simulink subsystem "Fault_Tolerant_Controller"  (R2022b)
settings: Solver=VariableStepAuto  StartTime=0.0  StopTime=10.0  RelTol=1e-3
libraries: matrix_library x2
settings Model: Creator=hunter  LastModifiedBy=hunter

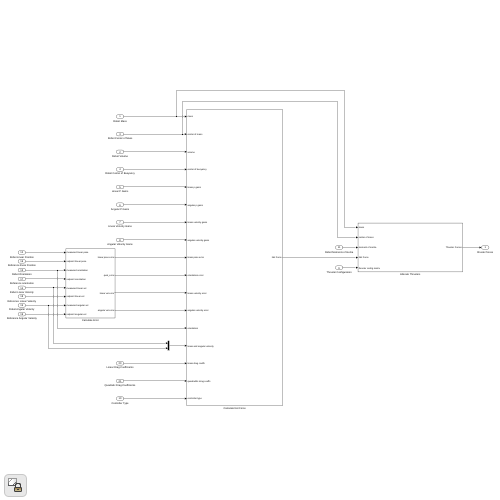
[thumbnail: Simulink's stored preview of the top-level diagram]
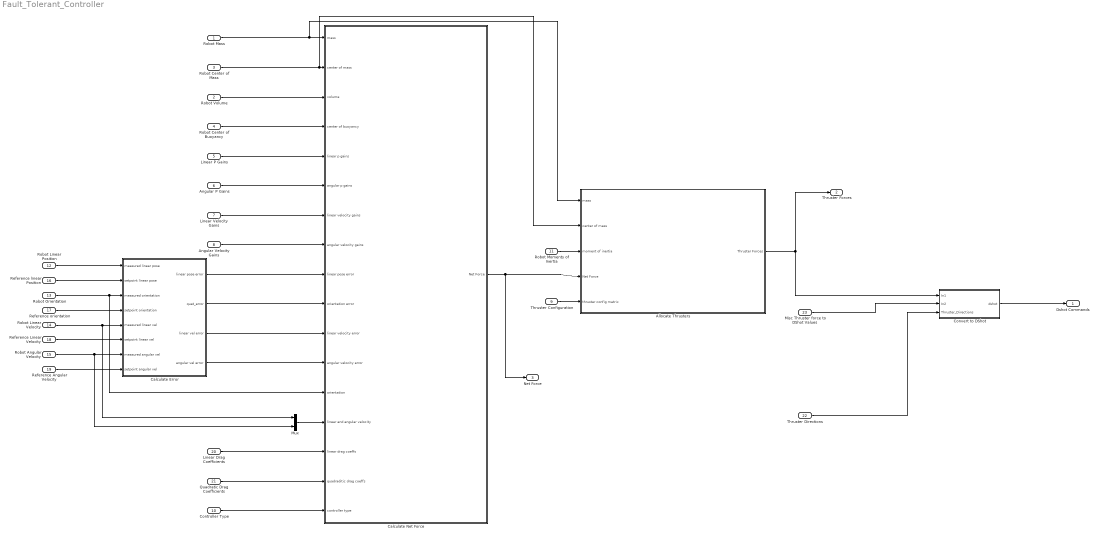
== system Fault_Tolerant_Controller ==
  Robot Mass : Inport  Unit=kg
  Robot Volume : Inport  Port=2  OutDataTypeStr=double
  Robot Center of Mass : Inport  Port=3  OutDataTypeStr=double  PortDimensions=[3 1]
  Robot Center of Buoyancy : Inport  Port=4  OutDataTypeStr=double  PortDimensions=[3 1]
  Linear P Gains : Inport  Port=5  OutDataTypeStr=double  PortDimensions=[3 3]
  Angular P Gains : Inport  Port=6  OutDataTypeStr=double  PortDimensions=[3 3]
  Linear Velocity Gains : Inport  Port=7  OutDataTypeStr=double  PortDimensions=[3 3]
  Angular Velocity Gains : Inport  Port=8  OutDataTypeStr=double  PortDimensions=[3 3]
  Thruster Configuration : Inport  Port=9  OutDataTypeStr=double  PortDimensions=[6 8]
  Controller Type : Inport  Port=10  OutDataTypeStr=boolean  PortDimensions=1
  Robot Moments of Inertia : Inport  Port=11  OutDataTypeStr=double  Unit=kg*m^2  PortDimensions=[3 1]
  Robot Linear Position : Inport  Port=12  OutDataTypeStr=double  PortDimensions=[3 1]
  Robot Orientation : Inport  Port=13  OutDataTypeStr=double  PortDimensions=[4 1]
  Robot Linear Velocity : Inport  Port=14  OutDataTypeStr=double  PortDimensions=[3 1]
  Robot Angular Velocity : Inport  Port=15  OutDataTypeStr=double  PortDimensions=[3 1]
  Reference linear Position : Inport  Port=16  OutDataTypeStr=double  PortDimensions=[3 1]
  Reference orientation : Inport  Port=17
  Reference Linear Velocity : Inport  Port=18
  Reference Angular Velocity : Inport  Port=19
  Linear Drag Coefficients : Inport  Port=20  OutDataTypeStr=double  PortDimensions=[6 1]
  Quadratic Drag Coefficients : Inport  Port=21  OutDataTypeStr=double  PortDimensions=[6 1]
  Thruster Directions : Inport  Port=22
  Misc Thruster force to DShot Values : Inport  Description=|  Port=23  OutDataTypeStr=double  PortDimensions=[11 1]
      | The rows of this column vector are defined as the following
      | Row 1 (C-style index 0): Max force for an individual thruster (max_force)
      | Row 2 (C-style index 1): Min force for and individual thruster (MIN_THRUST)
      | Row 3 (C-style index 2): Startup thrust force (STARTUP_THRUST)
      | 
      | Row 4 (C-style index 3): Positive slope for startup thrust (SU_THRUST.POS_SLOPE)
      | Row 5 (C-style index 4): Positive y-intercept for startup thrust (SU_THRUST.POS_YINT)
      | Row 6 (C-style index 5): Negative slope for startup thrust (SU_THRUST.NEG_SLOPE)
      | Row 7 (C-style index 6): Negative y-intercept for startup thrust (SU_THRUST.NEG_YINT)
      | 
      | Row 8 (C-style index 7): Positive slope for regular thrust (THRUST.POS_SLOPE)
      | Row 9 (C-style index 8): Positive y-intercept for regular thrust (THRUST.POS_YINT)
      | Row 10 (C-style index 9): Negative slope for regular thrust (THRUST.NEG_SLOPE)
      | Row 11 (C-style index 10): Negative y-intercept for regular thrust (THRUST.NEG_YINT)
      settings: AttributesFormatString=%<Description>
  Allocate Thrusters : Subsystem
  Calculate Error : Subsystem
  Calculate Net Force : Subsystem
  Convert to DShot : Subsystem
  Mux : Mux  Inputs=2
  Dshot Commands : Outport  OutDataTypeStr=int16  PortDimensions=[8 1]
  Thruster Forces : Outport  Port=2
  Net Force : Outport  Port=3
  wires:
  Robot Mass/1 -> Calculate Net Force/1(mass), Allocate Thrusters/1(mass)
  Robot Volume/1 -> Calculate Net Force/3(volume)
  Robot Center of Mass/1 -> Allocate Thrusters/2(center of mass), Calculate Net Force/2(center of mass)
  Robot Center of Buoyancy/1 -> Calculate Net Force/4(center of buoyancy)
  Linear P Gains/1 -> Calculate Net Force/5(linear p gains)
  Angular P Gains/1 -> Calculate Net Force/6(angular p gains)
  Linear Velocity Gains/1 -> Calculate Net Force/7(linear velocity gains)
  Angular Velocity Gains/1 -> Calculate Net Force/8(angular velocity gains)
  Controller Type/1 -> Calculate Net Force/17(controller type)
  Calculate Net Force/1(Net Force) -> Allocate Thrusters/4(Net Force), Net Force/1
  Thruster Configuration/1 -> Allocate Thrusters/5(thruster config matrix)
  Robot Moments of Inertia/1 -> Allocate Thrusters/3(moment of inertia)
  Robot Linear Position/1 -> Calculate Error/1(measured linear pose)
  Reference linear Position/1 -> Calculate Error/2(setpoint linear pose)
  Robot Orientation/1 -> Calculate Error/3(measured orientation), Calculate Net Force/13(orientation)
  Reference orientation/1 -> Calculate Error/4(setpoint orientation)
  Robot Linear Velocity/1 -> Calculate Error/5(measured linear vel), Mux/1
  Reference Linear Velocity/1 -> Calculate Error/6(setpoint linear vel)
  Robot Angular Velocity/1 -> Calculate Error/7(measured angular vel), Mux/2
  Reference Angular Velocity/1 -> Calculate Error/8(setpoint angular vel)
  Calculate Error/1(linear pose error) -> Calculate Net Force/9(linear pose error)
  Calculate Error/2(quat_error) -> Calculate Net Force/10(orientation error)
  Calculate Error/3(linear vel error) -> Calculate Net Force/11(linear velocity error)
  Calculate Error/4(angular vel error) -> Calculate Net Force/12(angular velocity error)
  Mux/1 -> Calculate Net Force/14(linear and angular velocity)
  Linear Drag Coefficients/1 -> Calculate Net Force/15(linear drag coeffs)
  Quadratic Drag Coefficients/1 -> Calculate Net Force/16(quadraditic drag coeffs)
  Allocate Thrusters/1(Thruster Forces) -> Convert to DShot/1(In1), Thruster Forces/1
  Misc Thruster force to DShot Values/1 -> Convert to DShot/2(In2)
  Thruster Directions/1 -> Convert to DShot/3(Thruster_Directions)
  Convert to DShot/1(dshot) -> Dshot Commands/1

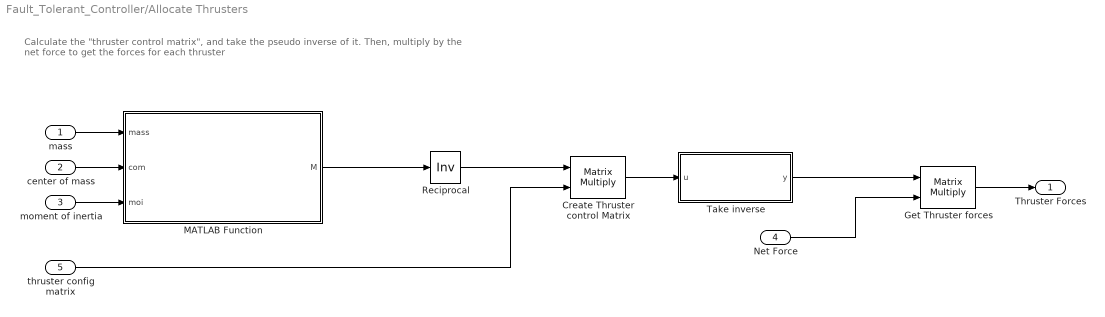
== system Fault_Tolerant_Controller/Allocate Thrusters ==
  note: Calculate the "thruster control matrix", and take the pseudo inverse of it.
      | Then, multiply by the net force to get the forces for each thruster
  mass : Inport
  center of mass : Inport  Port=2
  moment of inertia : Inport  Port=3
  Net Force : Inport  Port=4
  thruster config matrix : Inport  Port=5
  Create Thruster control Matrix : Product  Multiplication=Matrix(*)
  Get Thruster forces : Product  Multiplication=Matrix(*)
  MATLAB Function : MATLAB Function  TreatAsAtomicUnit=on
  Reciprocal : Product  Inputs=/  Multiplication=Matrix(*)
  Take inverse : MATLAB Function  TreatAsAtomicUnit=on
  Thruster Forces : Outport  OutDataTypeStr=double  PortDimensions=[8 1]
  wires:
  Get Thruster forces/1 -> Thruster Forces/1
  thruster config matrix/1 -> Create Thruster control Matrix/2
  Reciprocal/1 -> Create Thruster control Matrix/1
  Net Force/1 -> Get Thruster forces/2
  Take inverse/1(y) -> Get Thruster forces/1
  MATLAB Function/1(M) -> Reciprocal/1
  Create Thruster control Matrix/1 -> Take inverse/1(u)
  center of mass/1 -> MATLAB Function/2(com)
  moment of inertia/1 -> MATLAB Function/3(moi)
  mass/1 -> MATLAB Function/1(mass)

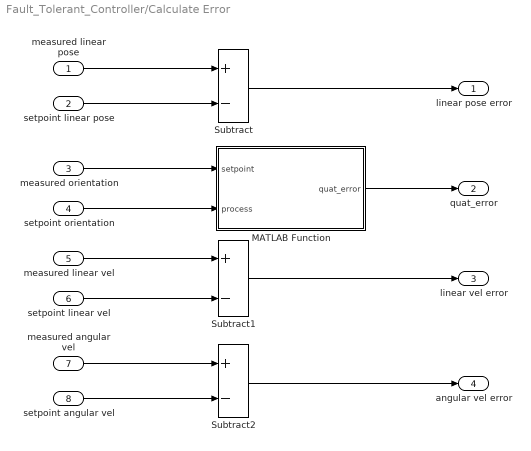
== system Fault_Tolerant_Controller/Calculate Error ==
  measured linear pose : Inport
  setpoint linear pose : Inport  Port=2
  measured orientation : Inport  Port=3
  setpoint orientation : Inport  Port=4  OutDataTypeStr=double  PortDimensions=[4 1]
  measured linear vel : Inport  Port=5
  setpoint linear vel : Inport  Port=6
  measured angular vel : Inport  Port=7
  setpoint angular vel : Inport  Port=8
  MATLAB Function : MATLAB Function  TreatAsAtomicUnit=on
  Subtract : Sum  Inputs=+-
  Subtract1 : Sum  Inputs=+-
  Subtract2 : Sum  Inputs=+-
  linear pose error : Outport
  quat_error : Outport  Port=2
  linear vel error : Outport  Port=3
  angular vel error : Outport  Port=4
  wires:
  setpoint angular vel/1 -> Subtract2/2
  measured angular vel/1 -> Subtract2/1
  measured linear vel/1 -> Subtract1/1
  setpoint linear vel/1 -> Subtract1/2
  setpoint linear pose/1 -> Subtract/2
  measured linear pose/1 -> Subtract/1
  Subtract/1 -> linear pose error/1
  Subtract1/1 -> linear vel error/1
  MATLAB Function/1(quat_error) -> quat_error/1
  Subtract2/1 -> angular vel error/1
  setpoint orientation/1 -> MATLAB Function/2(process)
  measured orientation/1 -> MATLAB Function/1(setpoint)

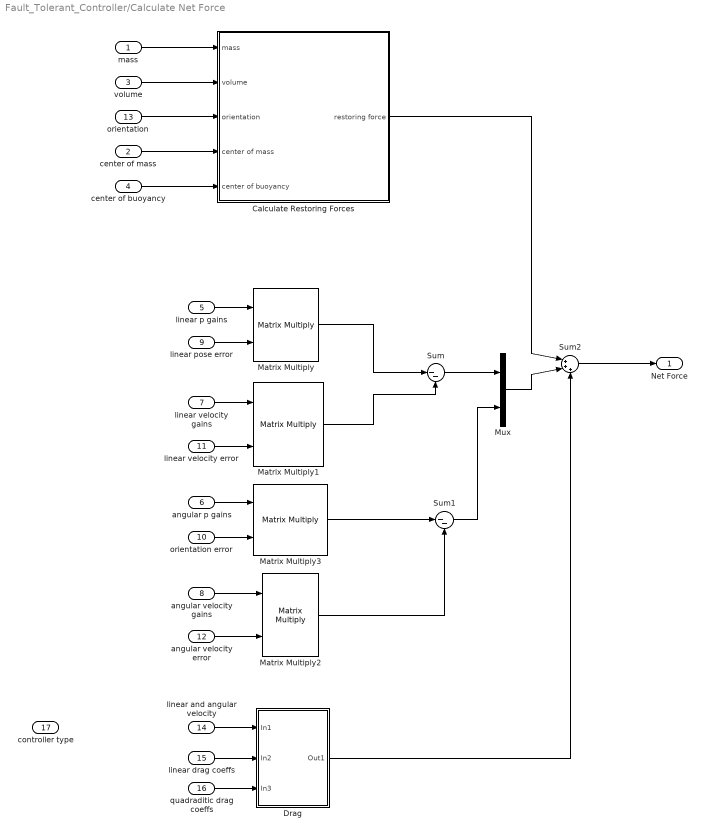
== system Fault_Tolerant_Controller/Calculate Net Force ==
  mass : Inport
  center of mass : Inport  Port=2
  volume : Inport  Port=3
  center of buoyancy : Inport  Port=4
  linear p gains : Inport  Port=5
  angular p gains : Inport  Port=6
  linear velocity gains : Inport  Port=7
  angular velocity gains : Inport  Port=8
  linear pose error : Inport  Port=9
  orientation error : Inport  Port=10
  linear velocity error : Inport  Port=11
  angular velocity error : Inport  Port=12
  orientation : Inport  Port=13
  linear and angular velocity : Inport  Port=14
  linear drag coeffs : Inport  Port=15
  quadraditic drag coeffs : Inport  Port=16
  controller type : Inport  Port=17
  Calculate Restoring Forces : Subsystem
  Drag : Subsystem
  Matrix Multiply{,1..3} (4 alike) : Product  Multiplication=Matrix(*)
  Mux : Mux  Inputs=2
  Sum : Sum  Inputs=|--
  Sum1 : Sum  Inputs=|--
  Sum2 : Sum  Inputs=|+++
  Net Force : Outport  OutDataTypeStr=double  Unit=N  PortDimensions=[6 1]
  wires:
  angular velocity gains/1 -> Matrix Multiply2/1
  angular velocity error/1 -> Matrix Multiply2/2
  angular p gains/1 -> Matrix Multiply3/1
  orientation error/1 -> Matrix Multiply3/2
  linear velocity gains/1 -> Matrix Multiply1/1
  linear velocity error/1 -> Matrix Multiply1/2
  linear pose error/1 -> Matrix Multiply/2
  linear p gains/1 -> Matrix Multiply/1
  Drag/1(Out1) -> Sum2/3
  quadraditic drag coeffs/1 -> Drag/3(In3)
  linear drag coeffs/1 -> Drag/2(In2)
  linear and angular velocity/1 -> Drag/1(In1)
  Calculate Restoring Forces/1(restoring force) -> Sum2/1
  Sum2/1 -> Net Force/1
  Mux/1 -> Sum2/2
  Sum1/1 -> Mux/2
  Matrix Multiply2/1 -> Sum1/2
  Matrix Multiply3/1 -> Sum1/1
  Matrix Multiply1/1 -> Sum/2
  Matrix Multiply/1 -> Sum/1
  center of buoyancy/1 -> Calculate Restoring Forces/5(center of buoyancy)
  center of mass/1 -> Calculate Restoring Forces/4(center of mass)
  orientation/1 -> Calculate Restoring Forces/3(orientation)
  volume/1 -> Calculate Restoring Forces/2(volume)
  mass/1 -> Calculate Restoring Forces/1(mass)
  Sum/1 -> Mux/1

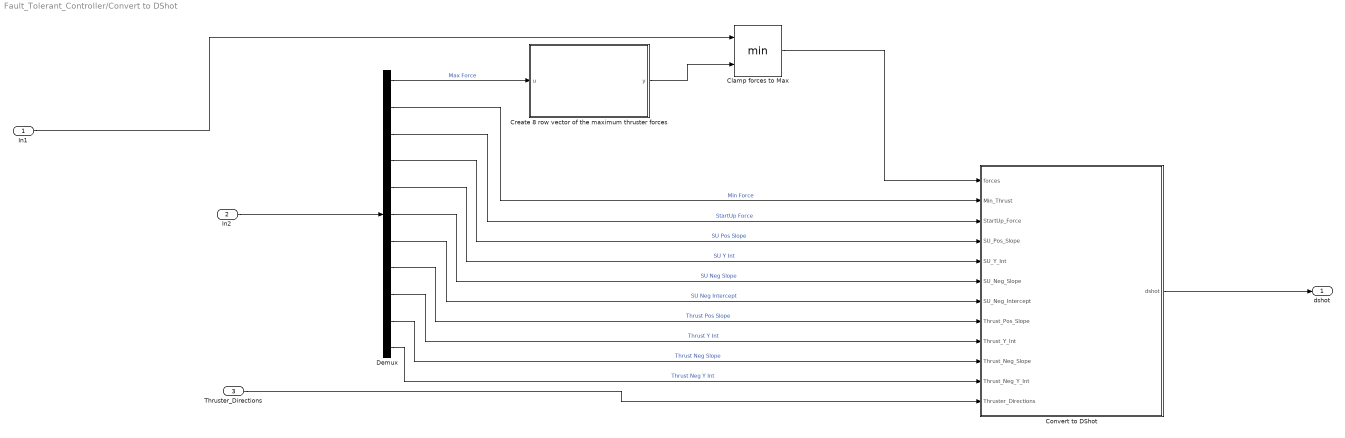
== system Fault_Tolerant_Controller/Convert to DShot ==
  In1 : Inport
  In2 : Inport  Port=2
  Thruster_Directions : Inport  Port=3
  Clamp forces to Max : MinMax  Inputs=2
  Convert to DShot : MATLAB Function  TreatAsAtomicUnit=on
  Create 8 row vector of the maximum thruster forces : MATLAB Function  TreatAsAtomicUnit=on
  Demux : Demux  Outputs=11
  dshot : Outport
  wires:
  Demux/7 -> Convert to DShot/7(SU_Neg_Intercept)  "SU Neg Intercept"
  Convert to DShot/1(dshot) -> dshot/1
  Demux/2 -> Convert to DShot/2(Min_Thrust)  "Min Force"
  Demux/8 -> Convert to DShot/8(Thrust_Pos_Slope)  "Thrust Pos Slope"
  Create 8 row vector of the maximum thruster forces/1(y) -> Clamp forces to Max/2
  Demux/1 -> Create 8 row vector of the maximum thruster forces/1(u)  "Max Force"
  Demux/10 -> Convert to DShot/10(Thrust_Neg_Slope)  "Thrust Neg Slope"
  Demux/5 -> Convert to DShot/5(SU_Y_Int)  "SU Y Int"
  Thruster_Directions/1 -> Convert to DShot/12(Thruster_Directions)
  Demux/11 -> Convert to DShot/11(Thrust_Neg_Y_Int)  "Thrust Neg Y Int"
  In1/1 -> Clamp forces to Max/1
  Demux/3 -> Convert to DShot/3(StartUp_Force)  "StartUp Force"
  Clamp forces to Max/1 -> Convert to DShot/1(forces)
  In2/1 -> Demux/1
  Demux/6 -> Convert to DShot/6(SU_Neg_Slope)  "SU Neg Slope"
  Demux/9 -> Convert to DShot/9(Thrust_Y_Int)  "Thrust Y Int"
  Demux/4 -> Convert to DShot/4(SU_Pos_Slope)  "SU Pos Slope"

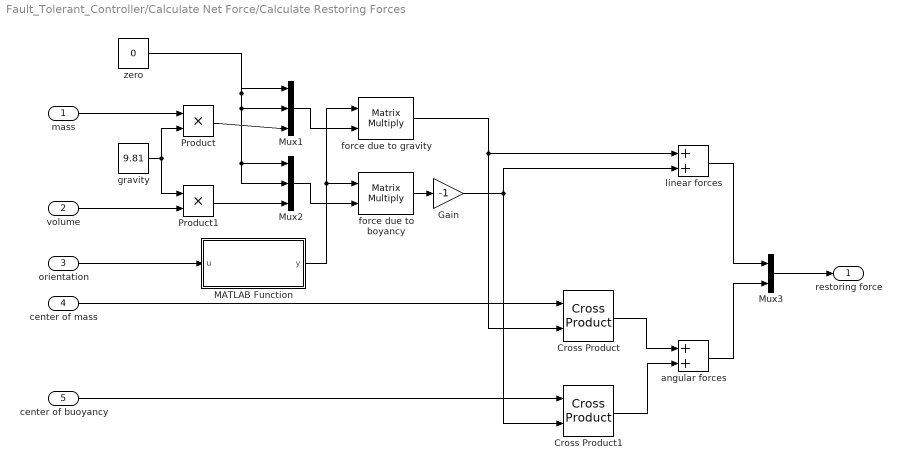
== system Fault_Tolerant_Controller/Calculate Net Force/Calculate Restoring Forces ==
  mass : Inport
  volume : Inport  Port=2
  orientation : Inport  Port=3
  center of mass : Inport  Port=4
  center of buoyancy : Inport  Port=5
  Cross Product : matrix_library/Cross Product
  Cross Product1 : matrix_library/Cross Product
  Gain : Gain  Gain=-1
  MATLAB Function : MATLAB Function  TreatAsAtomicUnit=on
  Mux1 : Mux  Inputs=3
  Mux2 : Mux  Inputs=3
  Mux3 : Mux  Inputs=2
  Product : Product
  Product1 : Product
  angular forces : Sum
  force due to boyancy : Product  Multiplication=Matrix(*)
  force due to gravity : Product  Multiplication=Matrix(*)
  gravity : Constant  Value=9.81  OutDataTypeStr=double
  linear forces : Sum
  zero : Constant  Value=0
  restoring force : Outport
  wires:
  Mux2/1 -> force due to boyancy/2
  Mux1/1 -> force due to gravity/2
  force due to gravity/1 -> linear forces/1, Cross Product/2
  Gain/1 -> linear forces/2, Cross Product1/2
  orientation/1 -> MATLAB Function/1(u)
  Cross Product/1 -> angular forces/1
  Product/1 -> Mux1/3
  force due to boyancy/1 -> Gain/1
  zero/1 -> Mux2/2, Mux2/1, Mux1/2, Mux1/1
  gravity/1 -> Product/2, Product1/1
  mass/1 -> Product/1
  center of buoyancy/1 -> Cross Product1/1
  angular forces/1 -> Mux3/2
  MATLAB Function/1(y) -> force due to gravity/1, force due to boyancy/1
  Mux3/1 -> restoring force/1
  center of mass/1 -> Cross Product/1
  volume/1 -> Product1/2
  linear forces/1 -> Mux3/1
  Cross Product1/1 -> angular forces/2
  Product1/1 -> Mux2/3

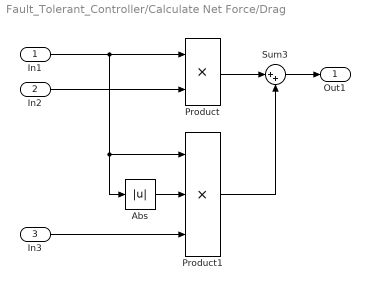
== system Fault_Tolerant_Controller/Calculate Net Force/Drag ==
  In1 : Inport
  In2 : Inport  Port=2
  In3 : Inport  Port=3
  Abs : Abs  SaturateOnIntegerOverflow=off
  Product : Product
  Product1 : Product  Inputs=3
  Sum3 : Sum  Inputs=|++
  Out1 : Outport
  wires:
  Sum3/1 -> Out1/1
  In2/1 -> Product/2
  In1/1 -> Abs/1, Product1/1, Product/1
  Product1/1 -> Sum3/2
  Abs/1 -> Product1/2
  In3/1 -> Product1/3
  Product/1 -> Sum3/1

== matlab function Fault_Tolerant_Controller/Allocate Thrusters/Take inverse ==
  data: u input; y output
function y = pseudo_inverse(u)
y = pinv(u);

== matlab function Fault_Tolerant_Controller/Allocate Thrusters/MATLAB Function ==
  data: mass input; com input; M output; moi input
% Create a 6x6 matrix representing the equations of motion for a rigid body
% Note that we only store the diagonals of the inertial tensor (I_xx, I_yy,
% and I_zz) in our robot yaml files.
%
% Taken from Fossen's Guidance and Control of Ocean Vehicles
%
function M = create_rigid_body_inertia_matrix(mass, com, moi)
m=mass;
c_x = com(1);
c_y = com(2);
c_z = com(3);

I_xx = moi(1);
I_yy = moi(2);
I_zz = moi(3);

M = [m      0       0       0       m*c_z   -m*c_y
     0      m       0       -m*c_z  0       m*c_x
     0      0       m       m*c_y   -m*c_x  0
     0      -m*c_z  m*c_y   I_xx    0       0
     m*c_z  0       -m*c_x  0       I_yy    0
     -m*c_y m*c_x   0       0       0       I_zz];

== matlab function Fault_Tolerant_Controller/Calculate Error/MATLAB Function ==
  data: setpoint input; quat_error output; process input
% Calculates the error between two quaternions
function quat_error = calc_quat_error(setpoint, process)
% quaternions are just row vectors, so doing transpose on the setpoint
% and process 
s_quat = transpose(setpoint); % quaternion(setpoint(1), setpoint(2), setpoint(3), setpoint(4));
p_quat = transpose(process); % quaternion(process(1), process(2), process(3), process(4));

err = quatmultiply(quatconj(s_quat), p_quat);

% Note that we only need the x y z terms of the quaternion error
% We also need it as a column vector to multiple it by the proprtional
% term matrix
quat_error = transpose(err(2:4));

== matlab function Fault_Tolerant_Controller/Calculate Net Force/Calculate Restoring Forces/MATLAB Function ==
  data: u input; y output
function y = quat_to_rot_mat(u)
% Note that quaternionis are just row vectors, so transposing u (a column
% vector), is all that is needed to turn it into a quaternion)
quat = quaternion(u(1), u(2), u(3), u(4));
y = quat2rotm(quat);

== matlab function Fault_Tolerant_Controller/Convert to DShot/Create 8 row vector of the maximum thruster forces ==
  data: u input; y output
function y = create_8_row_vector(u)

y = [u; u; u; u; u; u; u; u];

== matlab function Fault_Tolerant_Controller/Convert to DShot/Convert to DShot ==
  data: forces input; Min_Thrust input; StartUp_Force input; dshot output int16 size=[8 1]; SU_Pos_Slope input; SU_Y_Int input; SU_Neg_Slope input; SU_Neg_Intercept input; Thrust_Pos_Slope input; Thrust_Y_Int input; Thrust_Neg_Slope input; Thrust_Neg_Y_Int input; Thruster_Directions input
function dshot = convert_to_dshot(forces, Min_Thrust , StartUp_Force, SU_Pos_Slope, ...
    SU_Y_Int, SU_Neg_Slope, SU_Neg_Intercept, Thrust_Pos_Slope, ...
    Thrust_Y_Int, Thrust_Neg_Slope, Thrust_Neg_Y_Int, Thruster_Directions)

dshot = int16(zeros([8 1]));

for i = 1:8

    % no force is needed
    if abs(forces(i)) < Min_Thrust
        dshot(i) = int16(0);

    elseif forces(i) > 0 && forces(i) <= StartUp_Force
        if Thruster_Directions(i) == 0
            dshot(i) = int16(SU_Pos_Slope * forces(i) + SU_Y_Int);
        else
            dshot(i) = int16(-SU_Pos_Slope * forces(i) + SU_Neg_Intercept);
        end
    elseif forces(i) > 0 && forces(i) > StartUp_Force
        if Thruster_Directions(i) == 0
            dshot(i) = int16(Thrust_Pos_Slope * forces(i) + Thrust_Y_Int);
        else
            dshot(i) = int16(-Thrust_Pos_Slope * forces(i) + Thrust_Neg_Y_Int);
        end
    elseif forces(i) < 0 && forces(i) >= -StartUp_Force
        if Thruster_Directions(i) == 0
            dshot(i) = int16(SU_Neg_Slope * forces(i) + SU_Neg_Intercept);
        else
            dshot(i) = int16(-SU_Neg_Slope * forces(i) + SU_Y_Int);
        end
    elseif forces(i) < 0 && forces(i) < -StartUp_Force
        if Thruster_Directions(i) == 0
            dshot(i) = int16(Thrust_Neg_Slope * forces(i) + Thrust_Neg_Y_Int);
        else
            dshot(i) = int16(Thrust_Neg_Slope * forces(i) + Thrust_Y_Int);
        end
    else
        dshot(i) = int16(0);
    end
end
